simulink model "motor_feedback_test"  (R2018a)
settings: Solver=VariableStepAuto  StartTime=0.0  StopTime=10.0  RelTol=1e-3
libraries: motor_feedback x3
settings Model: Creator=vuwij  LastModifiedBy=vuwij

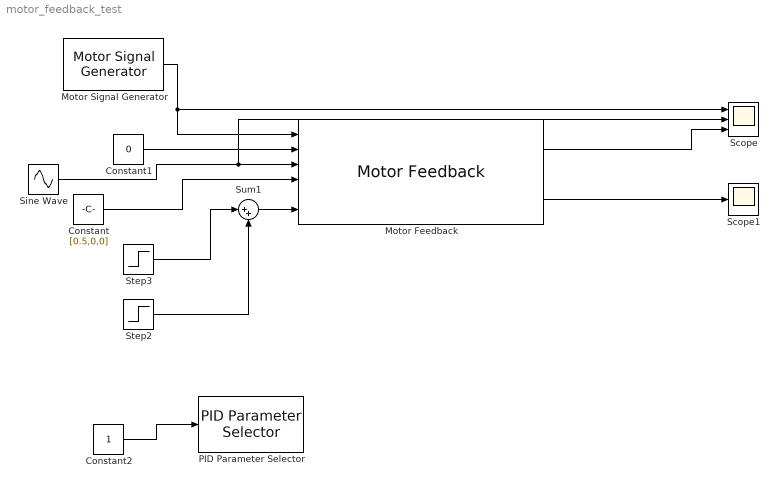
== system motor_feedback_test ==
  Constant : Constant  Value=[0.5,0,0]
  Constant1 : Constant  Value=0
  Constant2 : Constant
  Motor Feedback : motor_feedback/Motor Feedback  motorNumber=1  upperLimit=0.1  lowerLimit=-0.1  reverseDirection=on
  Motor Signal Generator : motor_feedback/Motor Signal Generator  SystemSampleTime=-1
  PID Parameter Selector : motor_feedback/PID Parameter Selector  pidParamSet=0  angleParamSet=motorFeedback.rightHipSideFront.pitch
  Scope : Scope  NumInputPorts=3
  Scope1 : Scope
  Sine Wave : Sin  Frequency=5  SampleTime=0.01
  Step2 : Step  Time=5  SampleTime=0
  Step3 : Step  Time=3  Before=1  After=0  SampleTime=0
  Sum1 : Sum  Inputs=|++
  wires:
  Constant/1 -> Motor Feedback/4
  Constant1/1 -> Motor Feedback/2
  Motor Feedback/1 -> Scope/3
  Motor Signal Generator/1 -> Motor Feedback/1, Scope/1
  Sum1/1 -> Motor Feedback/6
  Step2/1 -> Sum1/2
  Step3/1 -> Sum1/1
  Sine Wave/1 -> Motor Feedback/3, Scope/2
  Motor Feedback/2 -> Scope1/1
  Constant2/1 -> PID Parameter Selector/1
